simulink model "BootcampRobotModel"  (R2020b)
settings: Solver=VariableStepAuto  StartTime=0.0  StopTime=120  RelTol=1e-3
values from neighbouring files (symbols this model uses):
  A = [0, 0 ,1, 0 ... (first row only)    [BalancingRobotSystem.m]    (also in ControlBootcampModel.m = [0 1 0 0)
  B = [0; 0; 1/mc; 1/(L*mc)]    [BalancingRobotSystem.m]    (also in ControlBootcampModel.m = [0; 1/M; 0; s*1/(M*L)])
  C = [1 0 0 0]    [BalancingRobotSystem.m]    (also in ControlBootcampModel.m)
  K = acker(A,B, desiredPoles)    [BalancingRobotSystem.m]    (also in ControlBootcampModel.m = lqr(A,B,Q,R))
  x0 = [0; 5*pi/180; 0; 0;]    [BalancingRobotSystem.m]    (also in ControlBootcampModel.m = [0; 5*pi/180; 0; 0.5;])
settings Model: Creator=Nikola  LastModifiedBy=Nikola

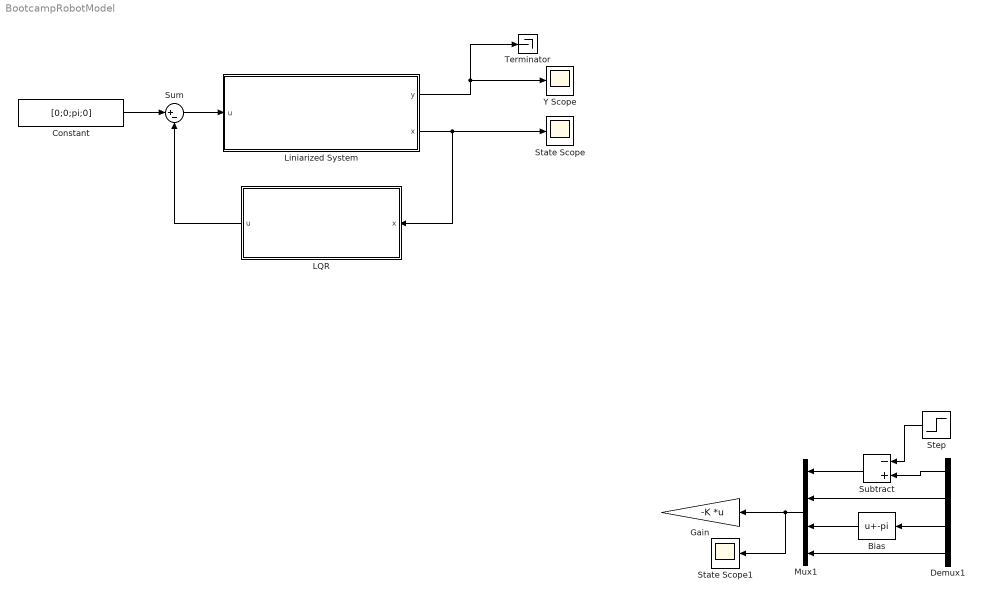
== system BootcampRobotModel ==
  Bias : Bias  Bias=-pi
  Constant : Constant  Value=[0;0;pi;0]
  Demux1 : Demux
  Gain : Gain  Gain=-K  Multiplication=Matrix(K*u) (u vector)
  LQR : Subsystem
  Liniarized System : Subsystem
  Mux1 : Mux
  State Scope : Scope
  State Scope1 : Scope
  Step : Step  Time=10  SampleTime=0
  Subtract : Sum  Inputs=-+
  Sum : Sum  Inputs=|+-
  Terminator : Terminator
  Y Scope : Scope
  wires:
  Liniarized System/1(y) -> Terminator/1, Y Scope/1
  Liniarized System/2(x) -> LQR/1(x), State Scope/1
  Demux1/1 -> Subtract/2
  Demux1/2 -> Mux1/2
  Demux1/3 -> Bias/1
  Subtract/1 -> Mux1/1
  Demux1/4 -> Mux1/4
  Bias/1 -> Mux1/3
  Step/1 -> Subtract/1
  Mux1/1 -> State Scope1/1, Gain/1
  Constant/1 -> Sum/1
  Sum/1 -> Liniarized System/1(u)
  LQR/1(u) -> Sum/2

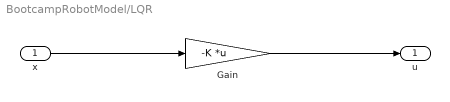
== system BootcampRobotModel/LQR ==
  x : Inport
  Gain : Gain  Gain=-K  Multiplication=Matrix(K*u)
  u : Outport
  wires:
  Gain/1 -> u/1
  x/1 -> Gain/1

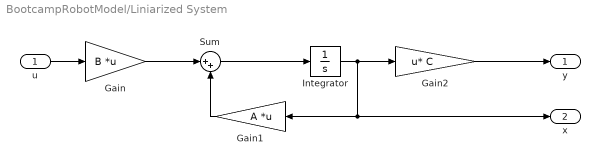
== system BootcampRobotModel/Liniarized System ==
  u : Inport
  Gain : Gain  Gain=B  Multiplication=Matrix(K*u)
  Gain1 : Gain  Gain=A  Multiplication=Matrix(K*u)
  Gain2 : Gain  Gain=C  Multiplication=Matrix(u*K)
  Integrator : Integrator  InitialCondition=x0
  Sum : Sum  Inputs=|++
  y : Outport
  x : Outport  Port=2
  wires:
  Integrator/1 -> Gain2/1, x/1, Gain1/1
  Gain/1 -> Sum/1
  Gain1/1 -> Sum/2
  Sum/1 -> Integrator/1
  u/1 -> Gain/1
  Gain2/1 -> y/1
